simulink model "lab_4_equalizer_lms_submatrix"  (R2012b)
settings: Solver=ode45  StartTime=0.0  StopTime=0.0011  RelTol=1e-3
values from neighbouring files (symbols this model uses):
  Ts = 1/Rs    (= 2.23214285714e-06)    [lab_4_parameters.m]
undefined symbols (not defined in the file or in its folder): D, dfilt, pskmod
libraries: dspsigops x3, commsink2 x3, dsparch4 x2, dspsnks4 x2, commdigbbndpm3 x2, dspsigattribs x1, dspspect3 x1, dspmisc x1, commeq2 x1, dspstat3 x1, commchan3 x1, commrandsrc2 x1
settings Model: Creator=yuw  LastModifiedBy=alex
settings OptimizationCC: InlineInvariantSignals=on  InitFltsAndDblsToZero=on
settings DebuggingCC: SaveWithParameterizedLinksMsg=none  SignalResolutionControl=TryResolveAllWithWarning  MultiTaskDSMMsg=warning  MultiTaskCondExecSysMsg=none  StrictBusMsg=None
settings RTWCC: IncludeERTFirstTime=on
settings GRTTargetCC: TargetFcnLib=ansi_tfl_tmw.mat  CombineOutputUpdateFcns=off  GRTInterface=on

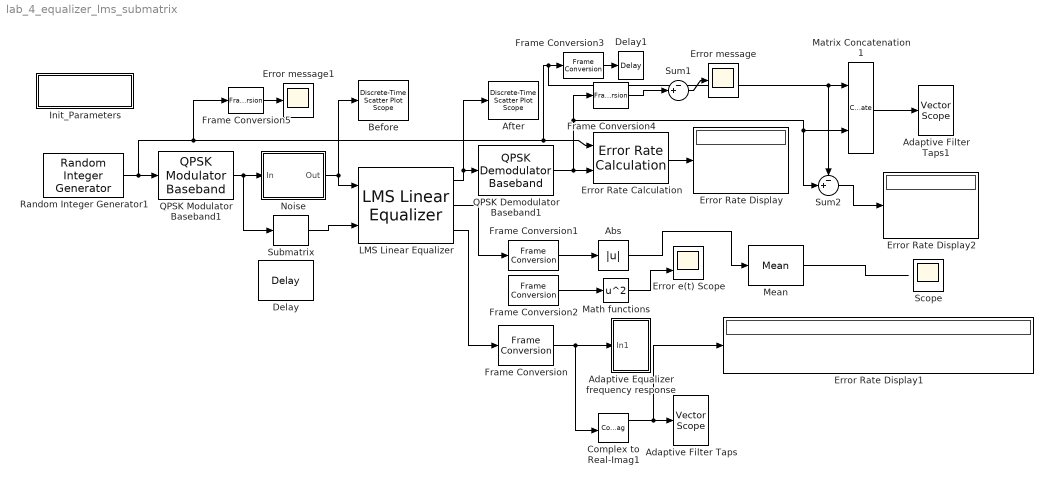
== system lab_4_equalizer_lms_submatrix ==
  Abs : Abs
  Adaptive Equalizer frequency response : Subsystem  AncestorBlock=dspsnks4/Spectrum Scope  DialogController=dspdialog.SpectrumScope  TreatAsAtomicUnit=on  SimViewingDevice=on  mask(Spectrum Scope){ScopeProperties=on, Domain=Frequency, HorizSpan=1, UseBuffer=off, BufferSize=128, Overlap=64, TreatMby1Signals=One channel, inpFftLenInherit=on, FFTlength=128, numAvg=2, DisplayProperties=off, AxisGrid=on, Memory=off, FrameNumber=on, AxisLegend=off, AxisZoom=off, OpenScopeAtSimStart=on, OpenScopeImmediately=off, FigPos=[8 424 450 170], AxisProperties=off, XUnits=Hertz, XRange=Two-sided ((-Fs/2...Fs/2]), XDisplay=0, InheritXIncr=off, XIncr=1e-5, XLabel=Samples, XLimit=Auto, YUnits=dBW/Hertz, XMax=1, XMin=0, YMin=-60.3983, YMax=-57.6842, YLabel=Magnitude-squared, dB, LineProperties=off, LineDisables=, LineStyles=--, LineMarkers=None, LineColors=[1 0 0], wintypeSpecScope=Hann, RsSpecScope=50, betaSpecScope=5, winsampSpecScope=Periodic, XAxisParamsVer=6.8, isFrameUpgraded=on}
      mask prompts: ScopeProperties "-------------------------------- Show scope properties ------------------------------------"; Domain "Input domain:"; HorizSpan "Time display span (number of frames):"; UseBuffer "Buffer input"; BufferSize "Buffer size:"; Overlap "Buffer overlap:"; TreatMby1Signals "Treat Mx1 and unoriented sample-based signals as:"; inpFftLenInherit "Specify FFT length"; FFTlength "FFT length:"; numAvg "Number of spectral averages:"; DisplayProperties "-------------------------------- Show display properties -----------------------------------"; AxisGrid "Show grid"; Memory "Persistence"; FrameNumber "Frame number"; AxisLegend "Channel legend"; AxisZoom "Compact display"; OpenScopeAtSimStart "Open scope at start of simulation"; OpenScopeImmediately "Open scope immediately"; FigPos "Scope position:"; AxisProperties "-------------------------------- Show axis properties ----------------------------------------"; XUnits "Frequency units:"; XRange "Spectrum type:"; XDisplay "Display DC as:"; InheritXIncr "Inherit sample increment from input"; XIncr "Sample time of original time series:"; XLabel "X-axis title:"; XLimit "X limits:"; YUnits "Spectrum units:"; XMax "X Max"; XMin "X Min"; YMin "Minimum Y-limit:"; YMax "Maximum Y-limit:"; YLabel "Y-axis title:"; LineProperties "-------------------------------- Show line properties -----------------------------------------"; LineDisables "Line visibility:"; LineStyles "Line styles:"; LineMarkers "Line markers:"; LineColors "Line colors:"; wintypeSpecScope "Window type:"; RsSpecScope "Stopband attenuation in dB:"; betaSpecScope "Beta:"; winsampSpecScope "Window sampling:"; XAxisParamsVer "Version of X-axis parameters:"; isFrameUpgraded "Frame upgraded:"
      mask help: Compute and display the mean-square spectrum or power spectral density of each input signal.
      mask init:
      | dspblkbfftscope2('setMaskEnables', ...
      |     UseBuffer, inpFftLenInherit, ...
      |     wintypeSpecScope, InheritXIncr);
      | [x,y,str] = dspblkbfftscope2('icon');
      | s = dspblkbfftscope2('init',YUnits, ...
      |     inpFftLenInherit, wintypeSpecScope, ...
      |     winsampSpecScope, InheritXIncr);
      settings: DeleteFcn=sdspfscope2([],[],[],'BlockDelete');  NameChangeFcn=sdspfscope2([],[],[],'NameChange');  RTWSystemCode=Function
      settings: CopyFcn=|
      | sdspfscope2([],[],[],'BlockCopy');
      | set_param(gcb,'XAxisParamsVer','6.9');
      | set_param(gcb,'isFrameUpgraded','on');
      mask Help: eval('blocksethelp');
      mask TypeOptions Domain: Time | Frequency | User-defined
      mask TypeOptions TreatMby1Signals: One channel | M channels
      mask TypeOptions XUnits: Hertz | rad/sec
      mask TypeOptions XRange: One-sided ([0...Fs/2]) | Two-sided ((-Fs/2...Fs/2]) | [0...Fs/2] | [-Fs/2...Fs/2] | [0...Fs]
      mask TypeOptions XLimit: Auto | User-defined
      mask TypeOptions YUnits: Watts/Hertz | Watts | dBW/Hertz | dBW | dBm/Hertz | dBm | Magnitude-squared | dB
      mask TypeOptions wintypeSpecScope: Bartlett | Blackman | Boxcar | Chebyshev | Hamming | Hann | Hanning | Kaiser | Triang
      mask TypeOptions winsampSpecScope: Symmetric | Periodic
      mask TypeOptions XAxisParamsVer: 6.8 | 6.9
      mask Display: plot(x,y); text(14,20,str);
  Adaptive Filter Taps : dspsnks4/Vector Scope  ScopeProperties=on  Domain=User-defined  HorizSpan=1  DisplayProperties=off  AxisGrid=on  Memory=off  FrameNumber=on  AxisLegend=off  AxisZoom=off  OpenScopeAtSimStart=on  OpenScopeImmediately=off  FigPos=[486 427 450 170]  AxisProperties=off  XUnits=Hertz  XRange=[0...Fs/2]  InheritXIncr=off  XIncr=1  XLabel=Coefficient Index  XLimit=Auto  XMin=0  XMax=1  XStart=0  YUnits=dB  YLabel=Amplitude  LineProperties=off  LineMarkers=.  XAxisParamsVer=6.8
      settings: YMin=-0.0861565175480312  YMax=0.95990385254224
  Adaptive Filter Taps1 : dspsnks4/Vector Scope  ScopeProperties=on  Domain=User-defined  HorizSpan=1  DisplayProperties=off  AxisGrid=on  Memory=off  FrameNumber=on  AxisLegend=off  AxisZoom=off  OpenScopeAtSimStart=off  OpenScopeImmediately=off  FigPos=[486 427 450 170]  AxisProperties=off  XUnits=Hertz  XRange=[0...Fs/2]  InheritXIncr=off  XIncr=1  XLabel=Coefficient Index  XLimit=Auto  XMin=0  XMax=1  XStart=0  YUnits=dB  YLabel=Amplitude  LineProperties=off  LineMarkers=.  XAxisParamsVer=6.8
      settings: YMin=-0.15  YMax=3.1575
  After : commsink2/Discrete-Time Scatter Plot Scope  Tag=ScatterPlot  sampPerSymb=1  offsetEye=0  numTraces=400  numNewFrames=10  LineMarkers=.  LineColors=b  fading=on  render=on  AxisGrid=on  xMin=-1.5  xMax=1.5  yMin=-1.5  yMax=1.5  inphaseLabel=In-phase Amplitude  quadratureLabel=Quadrature Amplitude  openScopeAtSimStart=on  FrameNumber=off  FigPos=[420 374 400 400]  figTitle=Scatter Plot  numLinesMax=8  block_type_=scatter
  Before : commsink2/Discrete-Time Scatter Plot Scope  Tag=ScatterPlot  sampPerSymb=1  offsetEye=0  numTraces=400  numNewFrames=10  LineMarkers=.  LineColors=b  fading=on  render=on  AxisGrid=on  xMin=-1.5  xMax=1.5  yMin=-1.5  yMax=1.5  inphaseLabel=In-phase Amplitude  quadratureLabel=Quadrature Amplitude  openScopeAtSimStart=on  FrameNumber=off  FigPos=[10 374 400 400]  figTitle=Scatter Plot  numLinesMax=8  block_type_=scatter
  Complex to Real-Imag1 : ComplexToRealImag
  Delay : dspsigops/Delay  InputProcessing=Inherited (this choice will be removed - see release notes)  dly_unit=Samples  delay=10  ic_detail=off  dif_ic_for_ch=off  dif_ic_for_dly=off  ic=0  reset_popup=None
  Delay1 : dspsigops/Delay  InputProcessing=Inherited (this choice will be removed - see release notes)  dly_unit=Samples  delay=4  ic_detail=off  dif_ic_for_ch=off  dif_ic_for_dly=off  ic=0  reset_popup=None
  Error Rate Calculation : commsink2/Error Rate Calculation  N=4  st_delay=0  cp_mode=Entire frame  subframe=[]  PMode=Port  WsName=ErrorVec  RsMode2=off  stop=off  numErr=100  maxBits=1e6
  Error Rate Display : Display
  Error Rate Display1 : Display
  Error Rate Display2 : Display
  Error e(t) Scope : Scope  NumInputPorts=2
      settings: TimeRange=6.400000000000001e-05  YMin=0.9682162866449512~-5  YMax=1.057816286644951~5  MaxDataPoints=10000
  Error message : Scope
      settings: TimeRange=1  YMin=-3  YMax=0  MaxDataPoints=10000
  Error message1 : Scope
      settings: TimeRange=1  YMin=-3  YMax=0  SaveName=ScopeData2  MaxDataPoints=10000
  Frame Conversion : FrameConversion
  Frame Conversion{1..5} (5 alike) : FrameConversion  OutFrame=Sample-based
  Init_Parameters : Subsystem
      settings: OpenFcn=lab_4_parameters
      mask Display: disp('lab_4_parameters')
  LMS Linear Equalizer : commeq2/LMS Linear  Equalizer  nTaps=4  nSamp=1  sigConst=pskmod([0:4-1],4)  delay=4  stepSize=0.01  leakage=1  initWeights=0  mode=off  outErr=on  outWeights=on
  Math functions : Math  Operator=square  SaturateOnIntegerOverflow=on
  Matrix Concatenation1 : Concatenate  Mode=Multidimensional array  ConcatenateDimension=2
  Mean : dspstat3/Mean  run=off  reset_popup=None  InputProcessing=Columns as channels (frame based)  directionMode=Each column  dimension=1  treatSBRowAsCol=on  roiEnable=off  roiType=Rectangles  roiPortion=Entire ROI  roiOutput=Individual statistics for each ROI  roiFlag=off  outputDataTypeStr=Inherit: Same as accumulator  outputLastDataTypeStr=Inherit: Same as accumulator  outputMin=[]  outputMax=[]  roundingMode=Floor  overflowMode=off
  Noise : Subsystem
  QPSK Demodulator Baseband1 : commdigbbndpm3/QPSK Demodulator Baseband  Ph=pi/4  Dec=Gray  OutType=Integer  DecType=Hard decision  VarSource=Dialog  Variance=1  outDtype1=Inherit via internal rule  outDtype2=Inherit via internal rule  derotateFactorWordLen=16
  QPSK Modulator Baseband1 : commdigbbndpm3/QPSK Modulator Baseband  InType=Integer  Enc=Gray  Ph=pi/4  outDtype=double  outWordLen=16  outUDDataType=sfix(16)  outFracLenMode=Best precision  outFracLen=15
  Random Integer Generator1 : commrandsrc2/Random Integer Generator  mul=4  seed=12345  Ts=Ts  frameBased=on  sampPerFrame=20  orient=off  outDataType=double
  Scope : Scope
      settings: Floating=on  YMin=-1.5  YMax=1.5  SaveName=ScopeData3
  Submatrix : dspmtrx3/Submatrix  RowSpan=Range of rows  RowStartMode=First  RowStartIndex=1  RowEndMode=Index  RowEndIndex=20  ColSpan=Range of columns  ColStartMode=First  ColStartIndex=1  ColEndMode=Last  ColEndIndex=1
  Sum1 : Sum  Inputs=-+|  SaturateOnIntegerOverflow=on  InputSameDT=on  OutDataTypeStr=Inherit: Same as first input
  Sum2 : Sum  Inputs=-+|  SaturateOnIntegerOverflow=on  InputSameDT=on  OutDataTypeStr=Inherit: Same as first input
  wires:
  Noise/1(Out) -> Before/1, LMS Linear Equalizer/1
  QPSK Modulator Baseband1/1 -> Noise/1(In), Submatrix/1
  Random Integer Generator1/1 -> QPSK Modulator Baseband1/1, Error Rate Calculation/1, Frame Conversion3/1, Matrix Concatenation1/1, Sum2/1, Frame Conversion5/1
  QPSK Demodulator Baseband1/1 -> Error Rate Calculation/2, Frame Conversion4/1, Matrix Concatenation1/2, Sum2/2
  Error Rate Calculation/1 -> Error Rate Display/1
  Frame Conversion/1 -> Adaptive Equalizer frequency response/1(In1), Complex to Real-Imag1/1
  Complex to Real-Imag1/1 -> Adaptive Filter Taps/1, Error Rate Display1/1
  Frame Conversion1/1 -> Abs/1
  Frame Conversion2/1 -> Math functions/1
  Sum1/1 -> Error message/1
  LMS Linear Equalizer/1 -> QPSK Demodulator Baseband1/1, After/1
  Frame Conversion3/1 -> Delay1/1
  Frame Conversion4/1 -> Sum1/2
  Frame Conversion5/1 -> Error message1/1
  LMS Linear Equalizer/2 -> Frame Conversion1/1
  LMS Linear Equalizer/3 -> Frame Conversion/1
  Matrix Concatenation1/1 -> Adaptive Filter Taps1/1
  Submatrix/1 -> LMS Linear Equalizer/2
  Sum2/1 -> Error Rate Display2/1
  Math functions/1 -> Error e(t) Scope/2
  Abs/1 -> Mean/1
  Mean/1 -> ?

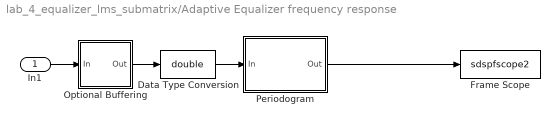
== system lab_4_equalizer_lms_submatrix/Adaptive Equalizer frequency response ==
  In1 : Inport
  Data Type Conversion : DataTypeConversion  OutDataTypeStr=double  SaturateOnIntegerOverflow=on  RndMeth=Zero
  Frame Scope : M-S-Function  FunctionName=sdspfscope2  Parameters=2  DisplayMFileStacktrace=off  mask(Frame Scope){}
      mask help: Level-2 MATLAB file S-function for frame scope.
      settings: CopyFcn=;
      mask Help: web(dspbhelp);
      mask Display: disp('Frame\nScope')
  Optional Buffering : Subsystem  mask(Replaceable Contents){oname=Buffer, osrc=dspbuff3/Buffer, oargs={'N','BufferSize','V','Overlap','ic','0','HasFrameUpgradeWarning','off'}, replace=strcmp(UseBuffer,'off')}
      mask prompts: oname "Relative name of blocks to replace:"; osrc "Simulink path to each source block:"; oargs "Parameter/value pairs to each block:"; replace "Replace with short-circuit:"
      mask help: Configurable subsystem holding blocks which may be replaced by virtual short-circuits (muxes) when not needed.
      mask init:
      | blk = gcb;
      | 
      | opts.name = oname; opts.src = osrc; opts.args = oargs;
      | dspskipblk(blk,opts,replace);
      | 
      | bufferBlk = [blk, '/Buffer'];
      | if strcmp(get_param(bufferBlk, 'BlockType'), 'Buffer')
      |     if strcmp(get_param(get_param(blk, 'parent'), 'TreatMby1Signals'), 'One channel');
      |         set_param(bufferBlk, 'TreatMby1Signals', 'One channel');
      |     else
      |         set_param(bufferBlk, 'TreatMby1Signals', 'M channels (this choice will be removed - see release notes)');
      |     end
      | end
  Periodogram : Subsystem  mask(Periodogram){measurement=Power spectral density, wintype=Hann, Rs=RsSpecScope, beta=betaSpecScope, winsamp=Periodic, FFTImplementation=Auto, inheritFFT=off, fftsize=FFTlength, navg=numAvg, inheritTs=off, Ts=XIncr}
      mask prompts: wintype "Window:"; Rs "Stopband attenuation in dB:"; winsamp "Window sampling:"; FFTImplementation "FFT implementation:"; inheritFFT "Inherit FFT length from input dimensions"; fftsize "FFT length:"; navg "Number of spectral averages:"; inheritTs "Inherit sample time from input"; Ts "Sample time of original time series:"
      mask help: Power spectral density and mean-square power spectrum estimation via the periodogram method and Welch's averaged, modified periodogram method.
      mask init:
      | [xe,x,y,iconStr]=dspblkshorttimefft2('icon',navg);
      | dspblkshorttimefft2('init',measurement,...
      |     inheritFFT,inheritTs,navg,Ts);
      mask Help: eval('blocksethelp');
      mask TypeOptions measurement: Power spectral density | Mean-square spectrum
      mask Callback measurement: dspblkshorttimefft2('dynamic');
      mask TypeOptions wintype: Bartlett | Blackman | Boxcar | Chebyshev | Hamming | Hann | Hanning | Kaiser | Triang
      mask Callback wintype: dspblkshorttimefft2('dynamic');
      mask TypeOptions winsamp: Symmetric | Periodic
      mask TypeOptions FFTImplementation: Auto | Radix-2 | FFTW
      mask Callback inheritFFT: dspblkshorttimefft2('dynamic');
      mask Callback inheritTs: dspblkshorttimefft2('dynamic');
      mask Display:
      | text(-3,1.15,iconStr);
      | plot((-xe),0,xe,1.3,x,y)
  wires:
  In1/1 -> Optional Buffering/1(In)
  Optional Buffering/1(Out) -> Data Type Conversion/1
  Data Type Conversion/1 -> Periodogram/1(In)
  Periodogram/1(Out) -> Frame Scope/1

== system lab_4_equalizer_lms_submatrix/Init_Parameters ==

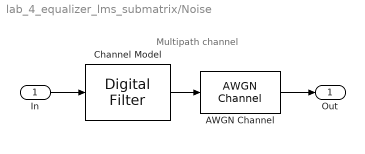
== system lab_4_equalizer_lms_submatrix/Noise ==
  note: Multipath channel
  In : Inport
  AWGN Channel : commchan3/AWGN Channel  InputProcessing=Inherited (this choice will be removed - see release notes)  seed=67  noiseMode="Signal to noise ratio  (SNR)"  EbNodB=EbNodB  EsNodB=10  SNRdB=40  bitsPerSym=1  Ps=1  Tsym=Ts  variance=1
  Channel Model : dsparch4/Digital Filter  TypePopup=FIR (all zeros)  IIRFiltStruct=Direct form I transposed  AllPoleFiltStruct=Direct form transposed  FIRFiltStruct=Direct form transposed  CoeffSource=Specify via dialog  NumCoeffs=[1 -.3 .1 .2j]  DenCoeffs=[1 0.1]  BiQuadCoeffs=[1 0.3 0.4 1 0.1 0.2]  LatticeCoeffs=[0.2 0.4]  denIgnore=on  FiltPerSampPopup=One filter per frame  IC=0  ICnum=0  ICden=0  roundingMode=Floor  overflowMode=off  ScaleValues=1  scaleValueFracLength=14  stageInFracLength=15  stageOutFracLength=15  FilterSource=Specify via dialog  dfiltObjectName=dfilt.dffir([1 2 1])  InputProcessing=Inherited (this choice will be removed - see release notes)
  Out : Outport
  wires:
  Channel Model/1 -> AWGN Channel/1
  AWGN Channel/1 -> Out/1
  In/1 -> Channel Model/1

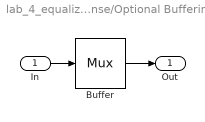
== system lab_4_equalizer_lms_submatrix/Adaptive Equalizer frequency response/Optional Buffering ==
  In : Inport
  Buffer : Mux  Inputs=1
  Out : Outport  InitialOutput=0
  wires:
  Buffer/1 -> Out/1
  In/1 -> Buffer/1

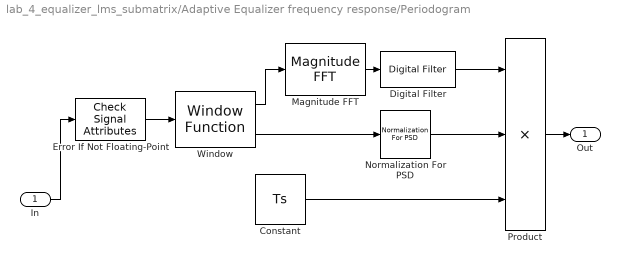
== system lab_4_equalizer_lms_submatrix/Adaptive Equalizer frequency response/Periodogram ==
  In : Inport
  Constant : Constant  Value=Ts  OutDataTypeStr=Inherit: Inherit via back propagation
  Digital Filter : dsparch4/Digital Filter  TypePopup=FIR (all zeros)  IIRFiltStruct=Direct form II transposed  AllPoleFiltStruct=Direct form  FIRFiltStruct=Direct form  CoeffSource=Specify via dialog  NumCoeffs=ones(navg,1)/navg  DenCoeffs=[1 0.1]  BiQuadCoeffs=[1 0.3 0.4 1 0.1 0.2]  LatticeCoeffs=[0.2 0.4]  denIgnore=on  FiltPerSampPopup=One filter per frame  IC=0  ICnum=0  ICden=0  roundingMode=Floor  overflowMode=off  ScaleValues=1  scaleValueFracLength=14  stageInFracLength=15  stageOutFracLength=15  FilterSource=Specify via dialog  dfiltObjectName=dfilt.dffir([1 2 1])
  Error If Not Floating-Point : dspsigattribs/Check Signal Attributes  SigAttribCheckMethod=Does not match attributes exactly  Complexity=Ignore  Frame=Ignore  DimsCheckMethod=Ignore  Dimensions=1-D  DatatypeCheckMethod=Is...  DatatypeGeneral=Floating-point  DtypeFloatSpecific=Any floating-point  DtypeFixedSpecific=Any fixed-point  DtypeIntSpecific=Any integer  SampleMode=Ignore
  Magnitude FFT : dspspect3/Magnitude FFT  mag_or_magsq=Magnitude squared  FFTImplementation=Auto  fftLenInherit=off  fftsize=fftsize
  Normalization For PSD : dspmisc/Normalization For PSD
  Product : Product  Inputs=***  SaturateOnIntegerOverflow=on  InputSameDT=on  OutDataTypeStr=Inherit: Same as first input
  Window : dspsigops/Window Function  winmode=Generate and apply window  wintype=Hann  sampmode=Continuous  samptime=1  N=64  Rs=Rs  beta=beta  winsamp=Periodic  UserWindow=hamming  OptParams=off  UserParams={1.0}  RowConvenienceOn=off  dataType=double  isSigned=on  wordLen=16  udDataType=sfix(16)  fracBitsMode=Best precision  numFracBits=15  roundingMode=Floor  overflowMode=off  numSidelobes=4  sidelobeLevel=-30
      settings: additionalParams=on
  Out : Outport  InitialOutput=0
  wires:
  In/1 -> Error If Not Floating-Point/1
  Magnitude FFT/1 -> Digital Filter/1
  Window/1 -> Magnitude FFT/1
  Product/1 -> Out/1
  Digital Filter/1 -> Product/1
  Normalization For PSD/1 -> Product/2
  Window/2 -> Normalization For PSD/1
  Error If Not Floating-Point/1 -> Window/1
  Constant/1 -> Product/3
